simulink model "controller"  (R2025b)
settings: Solver=VariableStepAuto  StartTime=0.0  StopTime=10.0  RelTol=1e-3
values from neighbouring files (symbols this model uses):
  Kd = 100.0    [controller.sldd]    (also in params.m = 100)
  Ki = 500.0    [controller.sldd]    (also in params.m = 500)
  Kp = 50.0    [controller.sldd]    (also in params.m = 50)
settings Model: DataDictionary=controller.sldd  Creator=mammadoo  LastModifiedBy=mammadoo

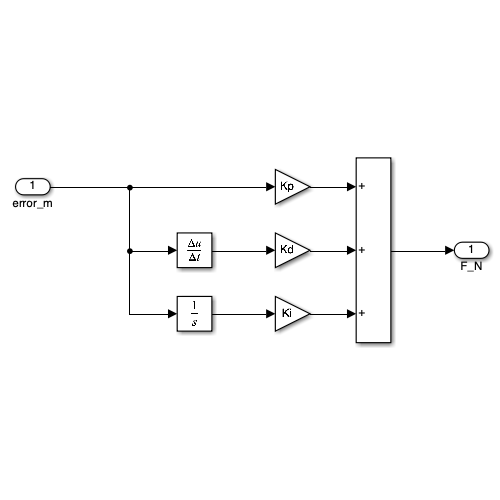
[thumbnail: Simulink's stored preview of the top-level diagram]
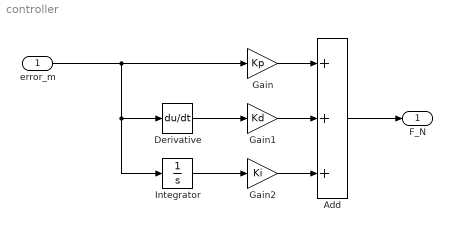
== system controller ==
  error_m : Inport
  Add : Sum  Inputs=+++
  Derivative : Derivative
  Gain : Gain  Gain=Kp
  Gain1 : Gain  Gain=Kd
  Gain2 : Gain  Gain=Ki
  Integrator : Integrator
  F_N : Outport
  wires:
  error_m/1 -> Integrator/1, Derivative/1, Gain/1
  Derivative/1 -> Gain1/1
  Integrator/1 -> Gain2/1
  Gain2/1 -> Add/3
  Gain1/1 -> Add/2
  Gain/1 -> Add/1
  Add/1 -> F_N/1
